simulink model "flightController"  (R2021a)
settings: Solver=ode3  StartTime=0  StopTime=10  FixedStep=Ts  RelTol=1e-3  EnableMultiTasking=on
undefined symbols (not defined in the file): Controller, ControlvsRed, D_ROLL, delays, DiscIntNeverNeededParam, g, I_ROLL, norm_act, Normalization, P_Pitch, P_ROLL, P_Roll, P_Yaw, P_z, PR_Start, save_time, sts_cnames, time_DisYaw, time_stepsX, time_stepsY, time_stepsZ, Ts, Vehicle, x0, x0_f
libraries: deeplib x5
(part 2 of 4)

== system flightController/Flight Controller/Perturbaciones/Perturbaciones en Pitch ==
  Add : Sum  Inputs=++++++++
  Pulse Generator1 : DiscretePulseGenerator  PulseType=Time based  Amplitude=P_Pitch(2)  Period=150  PulseWidth=0.01  PhaseDelay=time_stepsX(2)
  Pulse Generator2 : DiscretePulseGenerator  PulseType=Time based  Amplitude=P_Pitch(1)  Period=150  PulseWidth=0.02  PhaseDelay=time_stepsX(1)
  Pulse Generator3 : DiscretePulseGenerator  PulseType=Time based  Amplitude=P_Pitch(3)  Period=150  PulseWidth=0.01  PhaseDelay=time_stepsX(3)
  Pulse Generator4 : DiscretePulseGenerator  PulseType=Time based  Amplitude=P_Pitch(4)  Period=150  PulseWidth=0.01  PhaseDelay=time_stepsX(4)
  Pulse Generator5 : DiscretePulseGenerator  PulseType=Time based  Amplitude=P_Pitch(5)  Period=1500  PulseWidth=0.001  PhaseDelay=time_stepsX(5)
  Pulse Generator6 : DiscretePulseGenerator  PulseType=Time based  Amplitude=P_Pitch(6)  Period=150  PulseWidth=0.01  PhaseDelay=time_stepsX(6)
  Pulse Generator7 : DiscretePulseGenerator  PulseType=Time based  Amplitude=P_Pitch(7)  Period=1500  PulseWidth=0.001  PhaseDelay=time_stepsX(7)
  Pulse Generator8 : DiscretePulseGenerator  PulseType=Time based  Amplitude=P_Pitch(8)  Period=1500  PulseWidth=0.001  PhaseDelay=time_stepsX(8)
  Out1 : Outport
  wires:
  Pulse Generator2/1 -> Add/1
  Pulse Generator1/1 -> Add/2
  Pulse Generator3/1 -> Add/3
  Pulse Generator4/1 -> Add/4
  Pulse Generator5/1 -> Add/5
  Add/1 -> Out1/1
  Pulse Generator6/1 -> Add/6
  Pulse Generator7/1 -> Add/7
  Pulse Generator8/1 -> Add/8

== system flightController/Flight Controller/Perturbaciones/Perturbaciones en Roll ==
  Add : Sum  Inputs=++++++++
  Add1 : Sum  Commented=on  Inputs=+++++++
  Pulse Generator1 : DiscretePulseGenerator  PulseType=Time based  Amplitude=P_Roll(2)  Period=1500  PulseWidth=0.001  PhaseDelay=time_stepsY(2)
  Pulse Generator10 : DiscretePulseGenerator  Commented=on  PulseType=Time based  Amplitude=P_Roll(3)  Period=1500  PulseWidth=0.001  PhaseDelay=35
  Pulse Generator11 : DiscretePulseGenerator  Commented=on  PulseType=Time based  Amplitude=P_Roll(4)  Period=1500  PulseWidth=0.001  PhaseDelay=50
  Pulse Generator12 : DiscretePulseGenerator  Commented=on  PulseType=Time based  Amplitude=P_Roll(5)  Period=1500  PulseWidth=0.001  PhaseDelay=75
  Pulse Generator13 : DiscretePulseGenerator  Commented=on  PulseType=Time based  Amplitude=P_Roll(6)  Period=1500  PulseWidth=0.001  PhaseDelay=90
  Pulse Generator14 : DiscretePulseGenerator  Commented=on  PulseType=Time based  Amplitude=P_Roll(2)  Period=1500  PulseWidth=0.001  PhaseDelay=90
  Pulse Generator15 : DiscretePulseGenerator  PulseType=Time based  Amplitude=P_Roll(8)  Period=1500  PulseWidth=0.001  PhaseDelay=PR_Start
  Pulse Generator2 : DiscretePulseGenerator  PulseType=Time based  Amplitude=P_Roll(1)  Period=1500  PulseWidth=0.001  PhaseDelay=time_stepsY(1)
  Pulse Generator3 : DiscretePulseGenerator  PulseType=Time based  Amplitude=P_Roll(3)  Period=1500  PulseWidth=0.001  PhaseDelay=time_stepsY(3)
  Pulse Generator4 : DiscretePulseGenerator  PulseType=Time based  Amplitude=P_Roll(4)  Period=1500  PulseWidth=0.001  PhaseDelay=time_stepsY(4)
  Pulse Generator5 : DiscretePulseGenerator  PulseType=Time based  Amplitude=P_Roll(5)  Period=1500  PulseWidth=0.001  PhaseDelay=time_stepsY(5)
  Pulse Generator6 : DiscretePulseGenerator  PulseType=Time based  Amplitude=P_Roll(6)  Period=1500  PulseWidth=0.001  PhaseDelay=time_stepsY(6)
  Pulse Generator7 : DiscretePulseGenerator  PulseType=Time based  Amplitude=P_Roll(7)  Period=1500  PulseWidth=0.001  PhaseDelay=time_stepsY(7)
  Pulse Generator8 : DiscretePulseGenerator  Commented=on  PulseType=Time based  Amplitude=P_Roll(2)  Period=1500  PulseWidth=0.001  PhaseDelay=20
  Pulse Generator9 : DiscretePulseGenerator  Commented=on  PulseType=Time based  Amplitude=P_Roll(1)  Period=1500  PulseWidth=0.001  PhaseDelay=5
  Scope : Scope
  Out1 : Outport
  wires:
  Add/1 -> Out1/1
  Pulse Generator14/1 -> Add1/7
  Pulse Generator12/1 -> Add1/5
  Pulse Generator8/1 -> Add1/2
  Pulse Generator10/1 -> Add1/3
  Pulse Generator13/1 -> Add1/6
  Pulse Generator9/1 -> Add1/1
  Pulse Generator11/1 -> Add1/4
  Pulse Generator2/1 -> Add/2
  Pulse Generator1/1 -> Add/3
  Pulse Generator3/1 -> Add/4
  Pulse Generator4/1 -> Add/5
  Pulse Generator5/1 -> Add/6
  Pulse Generator6/1 -> Add/7
  Pulse Generator7/1 -> Add/8
  Pulse Generator15/1 -> Scope/1, Add/1

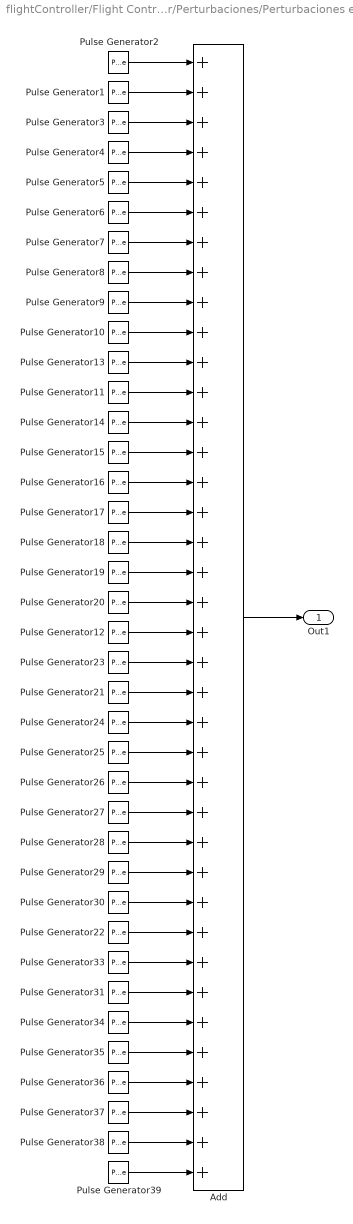
== system flightController/Flight Controller/Perturbaciones/Perturbaciones en Yaw ==
  Add : Sum  Inputs=++++++++++++++++++++++++++++++++++++++
  Pulse Generator1 : DiscretePulseGenerator  PulseType=Time based  Amplitude=P_Yaw(2)  Period=150  PulseWidth=0.01  PhaseDelay=time_DisYaw(2)
  Pulse Generator10 : DiscretePulseGenerator  PulseType=Time based  Amplitude=P_Yaw(10)  Period=1500  PulseWidth=0.001  PhaseDelay=time_DisYaw(10)
  Pulse Generator11 : DiscretePulseGenerator  PulseType=Time based  Amplitude=P_Yaw(12)  Period=150  PulseWidth=0.01  PhaseDelay=time_DisYaw(11)
  Pulse Generator12 : DiscretePulseGenerator  PulseType=Time based  Amplitude=P_Yaw(20)  Period=1500  PulseWidth=0.001  PhaseDelay=time_DisYaw(20)
  Pulse Generator13 : DiscretePulseGenerator  PulseType=Time based  Amplitude=P_Yaw(11)  Period=150  PulseWidth=0.02  PhaseDelay=time_DisYaw(11)
  Pulse Generator14 : DiscretePulseGenerator  PulseType=Time based  Amplitude=P_Yaw(13)  Period=150  PulseWidth=0.01  PhaseDelay=time_DisYaw(13)
  Pulse Generator15 : DiscretePulseGenerator  PulseType=Time based  Amplitude=P_Yaw(14)  Period=150  PulseWidth=0.01  PhaseDelay=time_DisYaw(14)
  Pulse Generator16 : DiscretePulseGenerator  PulseType=Time based  Amplitude=P_Yaw(15)  Period=1500  PulseWidth=0.001  PhaseDelay=time_DisYaw(15)
  Pulse Generator17 : DiscretePulseGenerator  PulseType=Time based  Amplitude=P_Yaw(16)  Period=150  PulseWidth=0.01  PhaseDelay=time_DisYaw(16)
  Pulse Generator18 : DiscretePulseGenerator  PulseType=Time based  Amplitude=P_Yaw(17)  Period=1500  PulseWidth=0.001  PhaseDelay=time_DisYaw(17)
  Pulse Generator19 : DiscretePulseGenerator  PulseType=Time based  Amplitude=P_Yaw(18)  Period=1500  PulseWidth=0.001  PhaseDelay=time_DisYaw(18)
  Pulse Generator2 : DiscretePulseGenerator  PulseType=Time based  Amplitude=P_Yaw(1)  Period=150  PulseWidth=0.02  PhaseDelay=time_DisYaw(1)
  Pulse Generator20 : DiscretePulseGenerator  PulseType=Time based  Amplitude=P_Yaw(19)  Period=1500  PulseWidth=0.001  PhaseDelay=time_DisYaw(19)
  Pulse Generator21 : DiscretePulseGenerator  PulseType=Time based  Amplitude=P_Yaw(22)  Period=150  PulseWidth=0.01  PhaseDelay=time_DisYaw(22)
  Pulse Generator22 : DiscretePulseGenerator  PulseType=Time based  Amplitude=P_Yaw(30)  Period=1500  PulseWidth=0.001  PhaseDelay=time_DisYaw(30)
  Pulse Generator23 : DiscretePulseGenerator  PulseType=Time based  Amplitude=P_Yaw(21)  Period=150  PulseWidth=0.02  PhaseDelay=time_DisYaw(21)
  Pulse Generator24 : DiscretePulseGenerator  PulseType=Time based  Amplitude=P_Yaw(23)  Period=150  PulseWidth=0.01  PhaseDelay=time_DisYaw(22)
  Pulse Generator25 : DiscretePulseGenerator  PulseType=Time based  Amplitude=P_Yaw(24)  Period=150  PulseWidth=0.01  PhaseDelay=time_DisYaw(24)
  Pulse Generator26 : DiscretePulseGenerator  PulseType=Time based  Amplitude=P_Yaw(25)  Period=1500  PulseWidth=0.001  PhaseDelay=time_DisYaw(25)
  Pulse Generator27 : DiscretePulseGenerator  PulseType=Time based  Amplitude=P_Yaw(26)  Period=150  PulseWidth=0.01  PhaseDelay=time_DisYaw(26)
  Pulse Generator28 : DiscretePulseGenerator  PulseType=Time based  Amplitude=P_Yaw(27)  Period=1500  PulseWidth=0.001  PhaseDelay=time_DisYaw(27)
  Pulse Generator29 : DiscretePulseGenerator  PulseType=Time based  Amplitude=P_Yaw(28)  Period=1500  PulseWidth=0.001  PhaseDelay=time_DisYaw(28)
  Pulse Generator3 : DiscretePulseGenerator  PulseType=Time based  Amplitude=P_Yaw(3)  Period=150  PulseWidth=0.01  PhaseDelay=time_DisYaw(3)
  Pulse Generator30 : DiscretePulseGenerator  PulseType=Time based  Amplitude=P_Yaw(29)  Period=1500  PulseWidth=0.001  PhaseDelay=time_DisYaw(29)
  Pulse Generator31 : DiscretePulseGenerator  PulseType=Time based  Amplitude=P_Yaw(32)  Period=150  PulseWidth=0.01  PhaseDelay=time_DisYaw(32)
  Pulse Generator33 : DiscretePulseGenerator  PulseType=Time based  Amplitude=P_Yaw(31)  Period=150  PulseWidth=0.02  PhaseDelay=time_DisYaw(31)
  Pulse Generator34 : DiscretePulseGenerator  PulseType=Time based  Amplitude=P_Yaw(33)  Period=150  PulseWidth=0.01  PhaseDelay=time_DisYaw(33)
  Pulse Generator35 : DiscretePulseGenerator  PulseType=Time based  Amplitude=P_Yaw(34)  Period=150  PulseWidth=0.01  PhaseDelay=time_DisYaw(34)
  Pulse Generator36 : DiscretePulseGenerator  PulseType=Time based  Amplitude=P_Yaw(35)  Period=1500  PulseWidth=0.001  PhaseDelay=time_DisYaw(35)
  Pulse Generator37 : DiscretePulseGenerator  PulseType=Time based  Amplitude=P_Yaw(36)  Period=150  PulseWidth=0.01  PhaseDelay=time_DisYaw(36)
  Pulse Generator38 : DiscretePulseGenerator  PulseType=Time based  Amplitude=P_Yaw(37)  Period=1500  PulseWidth=0.001  PhaseDelay=time_DisYaw(37)
  Pulse Generator39 : DiscretePulseGenerator  PulseType=Time based  Amplitude=P_Yaw(38)  Period=1500  PulseWidth=0.001  PhaseDelay=time_DisYaw(38)
  Pulse Generator4 : DiscretePulseGenerator  PulseType=Time based  Amplitude=P_Yaw(4)  Period=150  PulseWidth=0.01  PhaseDelay=time_DisYaw(4)
  Pulse Generator5 : DiscretePulseGenerator  PulseType=Time based  Amplitude=P_Yaw(5)  Period=1500  PulseWidth=0.001  PhaseDelay=time_DisYaw(5)
  Pulse Generator6 : DiscretePulseGenerator  PulseType=Time based  Amplitude=P_Yaw(6)  Period=150  PulseWidth=0.01  PhaseDelay=time_DisYaw(6)
  Pulse Generator7 : DiscretePulseGenerator  PulseType=Time based  Amplitude=P_Yaw(7)  Period=1500  PulseWidth=0.001  PhaseDelay=time_DisYaw(7)
  Pulse Generator8 : DiscretePulseGenerator  PulseType=Time based  Amplitude=P_Yaw(8)  Period=1500  PulseWidth=0.001  PhaseDelay=time_DisYaw(8)
  Pulse Generator9 : DiscretePulseGenerator  PulseType=Time based  Amplitude=P_Yaw(9)  Period=1500  PulseWidth=0.001  PhaseDelay=time_DisYaw(9)
  Out1 : Outport
  wires:
  Pulse Generator8/1 -> Add/8
  Pulse Generator7/1 -> Add/7
  Pulse Generator6/1 -> Add/6
  Add/1 -> Out1/1
  Pulse Generator5/1 -> Add/5
  Pulse Generator4/1 -> Add/4
  Pulse Generator3/1 -> Add/3
  Pulse Generator1/1 -> Add/2
  Pulse Generator2/1 -> Add/1
  Pulse Generator9/1 -> Add/9
  Pulse Generator10/1 -> Add/10
  Pulse Generator12/1 -> Add/20
  Pulse Generator13/1 -> Add/11
  Pulse Generator16/1 -> Add/15
  Pulse Generator11/1 -> Add/12
  Pulse Generator20/1 -> Add/19
  Pulse Generator19/1 -> Add/18
  Pulse Generator18/1 -> Add/17
  Pulse Generator15/1 -> Add/14
  Pulse Generator14/1 -> Add/13
  Pulse Generator17/1 -> Add/16
  Pulse Generator22/1 -> Add/30
  Pulse Generator23/1 -> Add/21
  Pulse Generator26/1 -> Add/25
  Pulse Generator21/1 -> Add/22
  Pulse Generator30/1 -> Add/29
  Pulse Generator29/1 -> Add/28
  Pulse Generator28/1 -> Add/27
  Pulse Generator25/1 -> Add/24
  Pulse Generator24/1 -> Add/23
  Pulse Generator27/1 -> Add/26
  Pulse Generator33/1 -> Add/31
  Pulse Generator36/1 -> Add/35
  Pulse Generator31/1 -> Add/32
  Pulse Generator39/1 -> Add/38
  Pulse Generator38/1 -> Add/37
  Pulse Generator35/1 -> Add/34
  Pulse Generator34/1 -> Add/33
  Pulse Generator37/1 -> Add/36

== system flightController/Flight Controller/Perturbaciones/Perturbaciones en Z ==
  Add : Sum  Inputs=++++++++++++++++++++
  Pulse Generator1 : DiscretePulseGenerator  PulseType=Time based  Amplitude=P_z(2)  Period=150  PulseWidth=0.5  PhaseDelay=time_stepsZ(2)
  Pulse Generator10 : DiscretePulseGenerator  PulseType=Time based  Amplitude=P_z(10)  Period=150  PulseWidth=0.5  PhaseDelay=time_stepsZ(10)
  Pulse Generator11 : DiscretePulseGenerator  PulseType=Time based  Amplitude=P_z(11)  Period=150  PulseWidth=0.5  PhaseDelay=time_stepsZ(11)
  Pulse Generator12 : DiscretePulseGenerator  PulseType=Time based  Amplitude=P_z(12)  Period=150  PulseWidth=0.5  PhaseDelay=time_stepsZ(12)
  Pulse Generator13 : DiscretePulseGenerator  PulseType=Time based  Amplitude=P_z(13)  Period=150  PulseWidth=0.5  PhaseDelay=time_stepsZ(13)
  Pulse Generator14 : DiscretePulseGenerator  PulseType=Time based  Amplitude=P_z(14)  Period=150  PulseWidth=0.5  PhaseDelay=time_stepsZ(14)
  Pulse Generator15 : DiscretePulseGenerator  PulseType=Time based  Amplitude=P_z(15)  Period=150  PulseWidth=0.5  PhaseDelay=time_stepsZ(15)
  Pulse Generator16 : DiscretePulseGenerator  PulseType=Time based  Amplitude=P_z(16)  Period=150  PulseWidth=0.2  PhaseDelay=time_stepsZ(16)
  Pulse Generator17 : DiscretePulseGenerator  PulseType=Time based  Amplitude=P_z(17)  Period=150  PulseWidth=0.3  PhaseDelay=time_stepsZ(17)
  Pulse Generator18 : DiscretePulseGenerator  PulseType=Time based  Amplitude=P_z(18)  Period=150  PulseWidth=0.1  PhaseDelay=time_stepsZ(18)
  Pulse Generator19 : DiscretePulseGenerator  PulseType=Time based  Amplitude=P_z(19)  Period=150  PulseWidth=0.5  PhaseDelay=time_stepsZ(19)
  Pulse Generator2 : DiscretePulseGenerator  PulseType=Time based  Amplitude=P_z(1)  Period=150  PulseWidth=0.5  PhaseDelay=time_stepsZ(1)
  Pulse Generator20 : DiscretePulseGenerator  PulseType=Time based  Amplitude=P_z(20)  Period=150  PulseWidth=0.01  PhaseDelay=time_stepsZ(20)
  Pulse Generator3 : DiscretePulseGenerator  PulseType=Time based  Amplitude=P_z(3)  Period=150  PulseWidth=0.5  PhaseDelay=time_stepsZ(3)
  Pulse Generator4 : DiscretePulseGenerator  PulseType=Time based  Amplitude=P_z(4)  Period=150  PulseWidth=0.5  PhaseDelay=time_stepsZ(4)
  Pulse Generator5 : DiscretePulseGenerator  PulseType=Time based  Amplitude=P_z(5)  Period=150  PulseWidth=0.5  PhaseDelay=time_stepsZ(5)
  Pulse Generator6 : DiscretePulseGenerator  PulseType=Time based  Amplitude=P_z(6)  Period=150  PulseWidth=0.5  PhaseDelay=time_stepsZ(6)
  Pulse Generator7 : DiscretePulseGenerator  PulseType=Time based  Amplitude=P_z(7)  Period=150  PulseWidth=0.5  PhaseDelay=time_stepsZ(7)
  Pulse Generator8 : DiscretePulseGenerator  PulseType=Time based  Amplitude=P_z(8)  Period=150  PulseWidth=0.5  PhaseDelay=time_stepsZ(8)
  Pulse Generator9 : DiscretePulseGenerator  PulseType=Time based  Amplitude=P_z(9)  Period=150  PulseWidth=0.5  PhaseDelay=time_stepsZ(9)
  Out1 : Outport
  wires:
  Pulse Generator2/1 -> Add/1
  Pulse Generator1/1 -> Add/2
  Pulse Generator3/1 -> Add/3
  Pulse Generator4/1 -> Add/4
  Pulse Generator5/1 -> Add/5
  Add/1 -> Out1/1
  Pulse Generator6/1 -> Add/6
  Pulse Generator7/1 -> Add/7
  Pulse Generator8/1 -> Add/8
  Pulse Generator9/1 -> Add/9
  Pulse Generator10/1 -> Add/10
  Pulse Generator11/1 -> Add/11
  Pulse Generator12/1 -> Add/12
  Pulse Generator13/1 -> Add/13
  Pulse Generator14/1 -> Add/14
  Pulse Generator15/1 -> Add/15
  Pulse Generator16/1 -> Add/16
  Pulse Generator17/1 -> Add/17
  Pulse Generator18/1 -> Add/18
  Pulse Generator19/1 -> Add/19
  Pulse Generator20/1 -> Add/20

== system flightController/Variant Subsystem/ANN/Subsystem ==
  Referencia : Inport
  Pos_estim : Inport  Port=2
  Sensores : Inport  Port=3  OutDataTypeStr=Bus: sensordata_t
  Math Function : Math  Commented=on  Operator=transpose  SaturateOnIntegerOverflow=on
  Mux : Mux  Inputs=5
  Subsystem : Subsystem
  Subsystem10 : Subsystem  Commented=on
  Subsystem11 : Subsystem  Commented=on
  Subsystem12 : Subsystem  Commented=on
  Subsystem13 : Subsystem
  Subsystem3 : Subsystem
  Norm_States : Outport
  wires:
  Mux/1 -> Norm_States/1
  Pos_estim/1 -> Subsystem13/1(In1)
  Subsystem13/1(Pos_Norm) -> Mux/1
  Referencia/1 -> Subsystem3/1(In1)
  Subsystem3/1(Z_r) -> Mux/2
  Subsystem3/2(Dz_r) -> Mux/3
  Sensores/1 -> Subsystem/1(In1)
  Subsystem13/2(Acceleracion Pos) -> Mux/5
  Subsystem/1(Ac_Dz) -> Mux/4

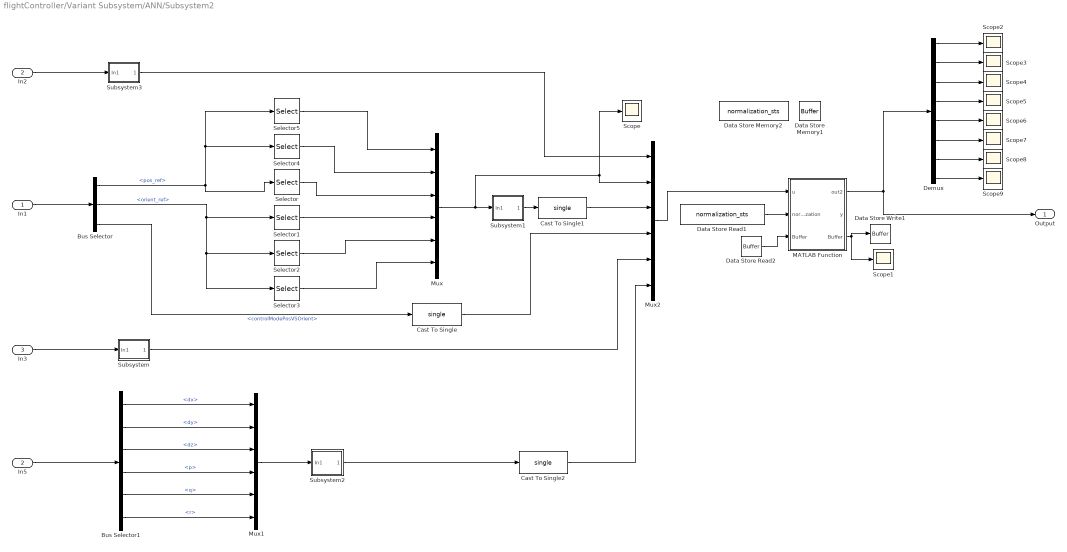
== system flightController/Variant Subsystem/ANN/Subsystem2 ==
  In1 : Inport
  In2 : Inport  Port=2
  In3 : Inport  Port=3
  Bus Selector : BusSelector  OutputSignals=pos_ref,orient_ref,controlModePosVSOrient
  Bus Selector1 : BusSelector  OutputSignals=dx,dy,dz,p,q,r
  Cast To Single : DataTypeConversion  OutDataTypeStr=single
  Cast To Single1 : DataTypeConversion  OutDataTypeStr=single
  Cast To Single2 : DataTypeConversion  OutDataTypeStr=single
  Data Store Memory1 : DataStoreMemory  DataStoreName=Buffer  ReadBeforeWriteMsg=warning  WriteAfterWriteMsg=warning  WriteAfterReadMsg=warning  InitialValue=repmat(x0,1,delays+1)  ShowAdditionalParam=off
  Data Store Memory2 : DataStoreMemory  DataStoreName=normalization_sts  ReadBeforeWriteMsg=warning  WriteAfterWriteMsg=warning  WriteAfterReadMsg=warning  InitialValue=normalization_sts  ShowAdditionalParam=off
  Data Store Read1 : DataStoreRead  DataStoreName=normalization_sts  IndexOptions=Index vector (dialog)  Indices=1  OutputSizes=1
  Data Store Read2 : DataStoreRead  DataStoreName=Buffer  IndexOptions=Index vector (dialog)  Indices=1  OutputSizes=1
  Data Store Write1 : DataStoreWrite  DataStoreName=Buffer  IndexOptions=Index vector (dialog)  Indices=1  OutputSizes=1
  Demux : Demux  Outputs=8
  In5 : InportShadow  Port=2
  MATLAB Function : MATLAB Function  TreatAsAtomicUnit=on
  Mux : Mux  Inputs=6
  Mux1 : Mux  Inputs=6
  Mux2 : Mux  Inputs=6
      settings: DisplayOption=signals
  Scope{,1..9} (10 alike) : Scope
  Selector : Selector  InputPortWidth=3  IndexOptions=Index vector (dialog)  Indices=[3]  OutputSizes=1
  Selector1 : Selector  InputPortWidth=3  IndexOptions=Index vector (dialog)  Indices=[1]  OutputSizes=1
  Selector2 : Selector  InputPortWidth=3  IndexOptions=Index vector (dialog)  Indices=[3]  OutputSizes=1
  Selector3 : Selector  InputPortWidth=3  IndexOptions=Index vector (dialog)  Indices=[2]  OutputSizes=1
  Selector4 : Selector  InputPortWidth=3  IndexOptions=Index vector (dialog)  Indices=[2]  OutputSizes=1
  Selector5 : Selector  InputPortWidth=3  IndexOptions=Index vector (dialog)  Indices=[1]  OutputSizes=1
  Subsystem : Subsystem
  Subsystem1 : Subsystem
  Subsystem2 : Subsystem
  Subsystem3 : Subsystem
  Output : Outport
  wires:
  In1/1 -> Bus Selector/1
  Bus Selector/2 -> Selector3/1, Selector2/1, Selector1/1  "<orient_ref>"
  Bus Selector/1 -> Selector/1, Selector5/1, Selector4/1  "<pos_ref>"
  Selector5/1 -> Mux/1
  Selector4/1 -> Mux/2
  Selector/1 -> Mux/3
  Selector1/1 -> Mux/4
  Selector2/1 -> Mux/5
  Selector3/1 -> Mux/6
  Mux/1 -> Mux2/2, Scope/1, Subsystem1/1(In1)
  In5/1 -> Bus Selector1/1
  Bus Selector1/1 -> Mux1/1  "<dx>"
  Bus Selector1/2 -> Mux1/2  "<dy>"
  Bus Selector1/3 -> Mux1/3  "<dz>"
  Bus Selector1/4 -> Mux1/4  "<p>"
  Bus Selector1/5 -> Mux1/5  "<q>"
  Bus Selector1/6 -> Mux1/6  "<r>"
  Mux1/1 -> Subsystem2/1(In1)
  Mux2/1 -> MATLAB Function/1(u)
  In3/1 -> Subsystem/1(In1)
  In2/1 -> Subsystem3/1(In1)
  Bus Selector/3 -> Cast To Single/1  "<controlModePosVSOrient>"
  Cast To Single1/1 -> Mux2/3
  Subsystem1/1(Out1) -> Cast To Single1/1
  Subsystem2/1(Out1) -> Cast To Single2/1
  Data Store Read1/1 -> MATLAB Function/2(normalization)
  Data Store Read2/1 -> MATLAB Function/3("Buffer ")
  MATLAB Function/3(Buffer) -> Data Store Write1/1, Scope1/1
  Subsystem3/1(Out5) -> Mux2/1
  Cast To Single2/1 -> Mux2/6
  Subsystem/1(Out5) -> Mux2/5
  Cast To Single/1 -> Mux2/4
  MATLAB Function/1(out2) -> Output/1, Demux/1
  Demux/1 -> Scope2/1
  Demux/2 -> Scope3/1
  Demux/3 -> Scope4/1
  Demux/4 -> Scope5/1
  Demux/5 -> Scope6/1
  Demux/6 -> Scope7/1
  Demux/7 -> Scope8/1
  Demux/8 -> Scope9/1

== system flightController/Variant Subsystem/ANN/Subsystem3 ==
  In1 : Inport
  Constant : Constant  Value=norm_act(1)
  Constant1 : Constant  Value=norm_act(3)
  Constant2 : Constant  Value=norm_act(5)
  Constant3 : Constant  Value=norm_act(7)
  Data Type Conversion : DataTypeConversion  OutDataTypeStr=single
  Demux : Demux
  Gain : Gain  Gain=(norm_act(2)-norm_act(1))  ParamDataTypeStr=single  OutDataTypeStr=single
  Gain1 : Gain  Gain=(norm_act(4)-norm_act(3))  OutDataTypeStr=single
  Gain2 : Gain  Gain=(norm_act(6)-norm_act(5))  OutDataTypeStr=single
  Gain3 : Gain  Gain=(norm_act(8)-norm_act(7))  OutDataTypeStr=single
  Mux : Mux
  Scope{,1..7} (8 alike) : Scope
  Sum{,1..3} (4 alike) : Sum  Inputs=|++
  motors_refout : Outport
  wires:
  In1/1 -> Demux/1
  Demux/4 -> Scope5/1, Gain3/1
  Constant/1 -> Sum/2
  Gain/1 -> Sum/1
  Demux/1 -> Scope4/1, Gain/1
  Gain1/1 -> Sum1/1
  Constant1/1 -> Sum1/2
  Demux/2 -> Gain1/1, Scope6/1
  Gain2/1 -> Sum2/1
  Constant2/1 -> Sum2/2
  Demux/3 -> Scope7/1, Gain2/1
  Gain3/1 -> Sum3/1
  Constant3/1 -> Sum3/2
  Mux/1 -> Data Type Conversion/1
  Data Type Conversion/1 -> motors_refout/1
  Sum3/1 -> Mux/4, Scope3/1
  Sum1/1 -> Mux/2, Scope1/1
  Sum/1 -> Mux/1, Scope/1
  Sum2/1 -> Mux/3, Scope2/1

== system flightController/Variant Subsystem/ANN/Subsystem4 ==
  In1 : Inport
  Constant : Constant  Value=norm_act(1)
  Constant1 : Constant  Value=norm_act(3)
  Constant2 : Constant  Value=norm_act(5)
  Constant3 : Constant  Value=norm_act(7)
  Data Type Conversion : DataTypeConversion  OutDataTypeStr=single
  Demux : Demux
  Gain : Gain  Gain=(norm_act(2)-norm_act(1))
  Gain1 : Gain  Gain=(norm_act(4)-norm_act(3))
  Gain2 : Gain  Gain=(norm_act(6)-norm_act(5))
  Gain3 : Gain  Gain=(norm_act(8)-norm_act(7))
  Mux : Mux
  Scope{,1..7} (8 alike) : Scope
  Sum{,1..3} (4 alike) : Sum  Inputs=|++
  motors_refout : Outport
  wires:
  In1/1 -> Demux/1
  Demux/4 -> Scope5/1, Gain3/1
  Constant/1 -> Sum/2
  Gain/1 -> Sum/1
  Demux/1 -> Scope4/1, Gain/1
  Gain1/1 -> Sum1/1
  Constant1/1 -> Sum1/2
  Demux/2 -> Gain1/1, Scope6/1
  Gain2/1 -> Sum2/1
  Constant2/1 -> Sum2/2
  Demux/3 -> Scope7/1, Gain2/1
  Gain3/1 -> Sum3/1
  Constant3/1 -> Sum3/2
  Mux/1 -> Data Type Conversion/1
  Data Type Conversion/1 -> motors_refout/1
  Sum3/1 -> Mux/4, Scope3/1
  Sum1/1 -> Mux/2, Scope1/1
  Sum/1 -> Mux/1, Scope/1
  Sum2/1 -> Mux/3, Scope2/1

== system flightController/Variant Subsystem/ANN_Feedback/Subsystem ==
  In1 : Inport
  Constant : Constant  Value=norm_act(1)
  Constant1 : Constant  Value=norm_act(3)
  Constant2 : Constant  Value=norm_act(5)
  Constant3 : Constant  Value=norm_act(7)
  Demux : Demux
  Gain1 : Gain  Gain=1/(norm_act(2)-norm_act(1))
  Gain2 : Gain  Gain=1/(norm_act(4)-norm_act(3))
  Gain3 : Gain  Gain=1/(norm_act(6)-norm_act(5))
  Gain4 : Gain  Gain=1/(norm_act(8)-norm_act(7))
  Mux : Mux
  Sum{,1..3} (4 alike) : Sum  Inputs=|+-
  Out1 : Outport
  wires:
  Sum/1 -> Gain1/1
  Demux/1 -> Sum/1
  Constant/1 -> Sum/2
  In1/1 -> Demux/1
  Sum1/1 -> Gain2/1
  Constant1/1 -> Sum1/2
  Demux/2 -> Sum1/1
  Demux/3 -> Sum2/1
  Constant2/1 -> Sum2/2
  Sum2/1 -> Gain3/1
  Sum3/1 -> Gain4/1
  Constant3/1 -> Sum3/2
  Demux/4 -> Sum3/1
  Mux/1 -> Out1/1
  Gain1/1 -> Mux/1
  Gain2/1 -> Mux/2
  Gain3/1 -> Mux/3
  Gain4/1 -> Mux/4

== system flightController/Variant Subsystem/ANN_Feedback/Subsystem1 ==
  Referencia : Inport
  Pos_estim : Inport  Port=2
  Sensores : Inport  Port=3  OutDataTypeStr=Bus: sensordata_t
  Math Function : Math  Commented=on  Operator=transpose  SaturateOnIntegerOverflow=on
  Mux : Mux
  Subsystem : Subsystem  Commented=on
  Subsystem10 : Subsystem  Commented=on
  Subsystem11 : Subsystem  Commented=on
  Subsystem12 : Subsystem  Commented=on
  Subsystem13 : Subsystem
  Subsystem3 : Subsystem
  Norm_States : Outport
  wires:
  Mux/1 -> Norm_States/1
  Pos_estim/1 -> Subsystem13/1(In1)
  Subsystem13/1(Pos_Norm) -> Mux/1
  Referencia/1 -> Subsystem3/1(In1)
  Subsystem3/1(Z_r) -> Mux/2
  Subsystem3/2(Dz_r) -> Mux/3
  Sensores/1 -> Subsystem/1(In1)
  Subsystem13/2(Acceleracion Pos) -> Mux/4

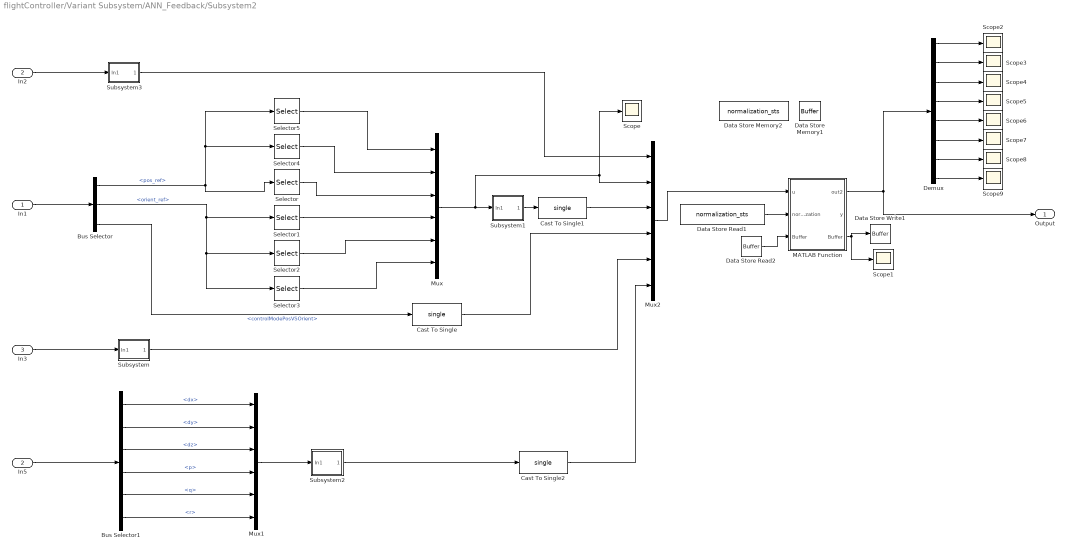
== system flightController/Variant Subsystem/ANN_Feedback/Subsystem2 ==
  In1 : Inport
  In2 : Inport  Port=2
  In3 : Inport  Port=3
  Bus Selector : BusSelector  OutputSignals=pos_ref,orient_ref,controlModePosVSOrient
  Bus Selector1 : BusSelector  OutputSignals=dx,dy,dz,p,q,r
  Cast To Single : DataTypeConversion  OutDataTypeStr=single
  Cast To Single1 : DataTypeConversion  OutDataTypeStr=single
  Cast To Single2 : DataTypeConversion  OutDataTypeStr=single
  Data Store Memory1 : DataStoreMemory  DataStoreName=Buffer  ReadBeforeWriteMsg=warning  WriteAfterWriteMsg=warning  WriteAfterReadMsg=warning  InitialValue=repmat(x0,1,delays+1)  ShowAdditionalParam=off
  Data Store Memory2 : DataStoreMemory  DataStoreName=normalization_sts  ReadBeforeWriteMsg=warning  WriteAfterWriteMsg=warning  WriteAfterReadMsg=warning  InitialValue=normalization_sts  ShowAdditionalParam=off
  Data Store Read1 : DataStoreRead  DataStoreName=normalization_sts  IndexOptions=Index vector (dialog)  Indices=1  OutputSizes=1
  Data Store Read2 : DataStoreRead  DataStoreName=Buffer  IndexOptions=Index vector (dialog)  Indices=1  OutputSizes=1
  Data Store Write1 : DataStoreWrite  DataStoreName=Buffer  IndexOptions=Index vector (dialog)  Indices=1  OutputSizes=1
  Demux : Demux  Outputs=8
  In5 : InportShadow  Port=2
  MATLAB Function : MATLAB Function  TreatAsAtomicUnit=on
  Mux : Mux  Inputs=6
  Mux1 : Mux  Inputs=6
  Mux2 : Mux  Inputs=6
      settings: DisplayOption=signals
  Scope{,1..9} (10 alike) : Scope
  Selector : Selector  InputPortWidth=3  IndexOptions=Index vector (dialog)  Indices=[3]  OutputSizes=1
  Selector1 : Selector  InputPortWidth=3  IndexOptions=Index vector (dialog)  Indices=[1]  OutputSizes=1
  Selector2 : Selector  InputPortWidth=3  IndexOptions=Index vector (dialog)  Indices=[3]  OutputSizes=1
  Selector3 : Selector  InputPortWidth=3  IndexOptions=Index vector (dialog)  Indices=[2]  OutputSizes=1
  Selector4 : Selector  InputPortWidth=3  IndexOptions=Index vector (dialog)  Indices=[2]  OutputSizes=1
  Selector5 : Selector  InputPortWidth=3  IndexOptions=Index vector (dialog)  Indices=[1]  OutputSizes=1
  Subsystem : Subsystem
  Subsystem1 : Subsystem
  Subsystem2 : Subsystem
  Subsystem3 : Subsystem
  Output : Outport
  wires:
  In1/1 -> Bus Selector/1
  Bus Selector/2 -> Selector3/1, Selector2/1, Selector1/1  "<orient_ref>"
  Bus Selector/1 -> Selector/1, Selector5/1, Selector4/1  "<pos_ref>"
  Selector5/1 -> Mux/1
  Selector4/1 -> Mux/2
  Selector/1 -> Mux/3
  Selector1/1 -> Mux/4
  Selector2/1 -> Mux/5
  Selector3/1 -> Mux/6
  Mux/1 -> Mux2/2, Scope/1, Subsystem1/1(In1)
  In5/1 -> Bus Selector1/1
  Bus Selector1/1 -> Mux1/1  "<dx>"
  Bus Selector1/2 -> Mux1/2  "<dy>"
  Bus Selector1/3 -> Mux1/3  "<dz>"
  Bus Selector1/4 -> Mux1/4  "<p>"
  Bus Selector1/5 -> Mux1/5  "<q>"
  Bus Selector1/6 -> Mux1/6  "<r>"
  Mux1/1 -> Subsystem2/1(In1)
  Mux2/1 -> MATLAB Function/1(u)
  In3/1 -> Subsystem/1(In1)
  In2/1 -> Subsystem3/1(In1)
  Bus Selector/3 -> Cast To Single/1  "<controlModePosVSOrient>"
  Cast To Single1/1 -> Mux2/3
  Subsystem1/1(Out1) -> Cast To Single1/1
  Subsystem2/1(Out1) -> Cast To Single2/1
  Data Store Read1/1 -> MATLAB Function/2(normalization)
  Data Store Read2/1 -> MATLAB Function/3("Buffer ")
  MATLAB Function/3(Buffer) -> Data Store Write1/1, Scope1/1
  Subsystem3/1(Out5) -> Mux2/1
  Cast To Single2/1 -> Mux2/6
  Subsystem/1(Out5) -> Mux2/5
  Cast To Single/1 -> Mux2/4
  Demux/1 -> Scope2/1
  Demux/2 -> Scope3/1
  Demux/3 -> Scope4/1
  Demux/4 -> Scope5/1
  Demux/5 -> Scope6/1
  Demux/6 -> Scope7/1
  Demux/7 -> Scope8/1
  Demux/8 -> Scope9/1
  MATLAB Function/1(out2) -> Output/1, Demux/1

== system flightController/Variant Subsystem/ANN_Feedback/Subsystem4 ==
  In1 : Inport
  Constant : Constant  Value=norm_act(1)
  Constant1 : Constant  Value=norm_act(3)
  Constant2 : Constant  Value=norm_act(5)
  Constant3 : Constant  Value=norm_act(7)
  Data Type Conversion : DataTypeConversion  OutDataTypeStr=single
  Demux : Demux
  Gain : Gain  Gain=(norm_act(2)-norm_act(1))
  Gain1 : Gain  Gain=(norm_act(4)-norm_act(3))
  Gain2 : Gain  Gain=(norm_act(6)-norm_act(5))
  Gain3 : Gain  Gain=(norm_act(8)-norm_act(7))
  Mux : Mux
  Scope{,1..7} (8 alike) : Scope
  Sum{,1..3} (4 alike) : Sum  Inputs=|++
  motors_refout : Outport
  wires:
  Sum2/1 -> Scope2/1, Mux/3
  Sum/1 -> Scope/1, Mux/1
  Sum1/1 -> Scope1/1, Mux/2
  Sum3/1 -> Scope3/1, Mux/4
  Data Type Conversion/1 -> motors_refout/1
  Mux/1 -> Data Type Conversion/1
  Constant3/1 -> Sum3/2
  Gain3/1 -> Sum3/1
  Demux/3 -> Gain2/1, Scope7/1
  Constant2/1 -> Sum2/2
  Gain2/1 -> Sum2/1
  Demux/2 -> Scope6/1, Gain1/1
  Constant1/1 -> Sum1/2
  Gain1/1 -> Sum1/1
  Demux/1 -> Gain/1, Scope4/1
  Gain/1 -> Sum/1
  Constant/1 -> Sum/2
  Demux/4 -> Gain3/1, Scope5/1
  In1/1 -> Demux/1

== system flightController/Variant Subsystem/ANN_Feedback/Subsystem5 ==
  In1 : Inport
  Constant : Constant  Value=norm_act(1)
  Constant1 : Constant  Value=norm_act(3)
  Constant2 : Constant  Value=norm_act(5)
  Constant3 : Constant  Value=norm_act(7)
  Data Type Conversion : DataTypeConversion  OutDataTypeStr=single
  Demux : Demux
  Gain : Gain  Gain=(norm_act(2)-norm_act(1))
  Gain1 : Gain  Gain=(norm_act(4)-norm_act(3))
  Gain2 : Gain  Gain=(norm_act(6)-norm_act(5))
  Gain3 : Gain  Gain=(norm_act(8)-norm_act(7))
  Mux : Mux
  Scope{,1..7} (8 alike) : Scope
  Sum{,1..3} (4 alike) : Sum  Inputs=|++
  motors_refout : Outport
  wires:
  In1/1 -> Demux/1
  Demux/4 -> Scope5/1, Gain3/1
  Constant/1 -> Sum/2
  Gain/1 -> Sum/1
  Demux/1 -> Scope4/1, Gain/1
  Gain1/1 -> Sum1/1
  Constant1/1 -> Sum1/2
  Demux/2 -> Gain1/1, Scope6/1
  Gain2/1 -> Sum2/1
  Constant2/1 -> Sum2/2
  Demux/3 -> Scope7/1, Gain2/1
  Gain3/1 -> Sum3/1
  Constant3/1 -> Sum3/2
  Mux/1 -> Data Type Conversion/1
  Data Type Conversion/1 -> motors_refout/1
  Sum3/1 -> Mux/4, Scope3/1
  Sum1/1 -> Mux/2, Scope1/1
  Sum/1 -> Mux/1, Scope/1
  Sum2/1 -> Mux/3, Scope2/1

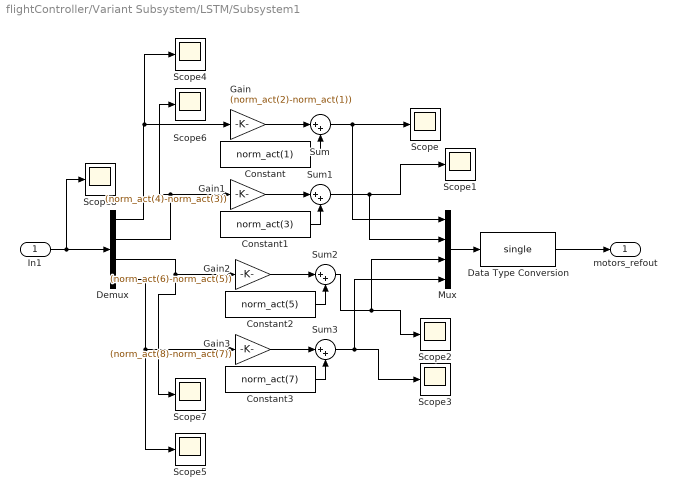
== system flightController/Variant Subsystem/LSTM/Subsystem1 ==
  In1 : Inport
  Constant : Constant  Value=norm_act(1)
  Constant1 : Constant  Value=norm_act(3)
  Constant2 : Constant  Value=norm_act(5)
  Constant3 : Constant  Value=norm_act(7)
  Data Type Conversion : DataTypeConversion  OutDataTypeStr=single
  Demux : Demux
  Gain : Gain  Gain=(norm_act(2)-norm_act(1))
  Gain1 : Gain  Gain=(norm_act(4)-norm_act(3))
  Gain2 : Gain  Gain=(norm_act(6)-norm_act(5))
  Gain3 : Gain  Gain=(norm_act(8)-norm_act(7))
  Mux : Mux
  Scope{,1..8} (9 alike) : Scope
  Sum{,1..3} (4 alike) : Sum  Inputs=|++
  motors_refout : Outport
  wires:
  In1/1 -> Scope8/1, Demux/1
  Demux/4 -> Scope5/1, Gain3/1
  Constant/1 -> Sum/2
  Gain/1 -> Sum/1
  Demux/1 -> Scope4/1, Gain/1
  Gain1/1 -> Sum1/1
  Constant1/1 -> Sum1/2
  Demux/2 -> Gain1/1, Scope6/1
  Gain2/1 -> Sum2/1
  Constant2/1 -> Sum2/2
  Demux/3 -> Scope7/1, Gain2/1
  Gain3/1 -> Sum3/1
  Constant3/1 -> Sum3/2
  Mux/1 -> Data Type Conversion/1
  Data Type Conversion/1 -> motors_refout/1
  Sum3/1 -> Mux/4, Scope3/1
  Sum1/1 -> Mux/2, Scope1/1
  Sum2/1 -> Mux/3, Scope2/1
  Sum/1 -> Mux/1, Scope/1

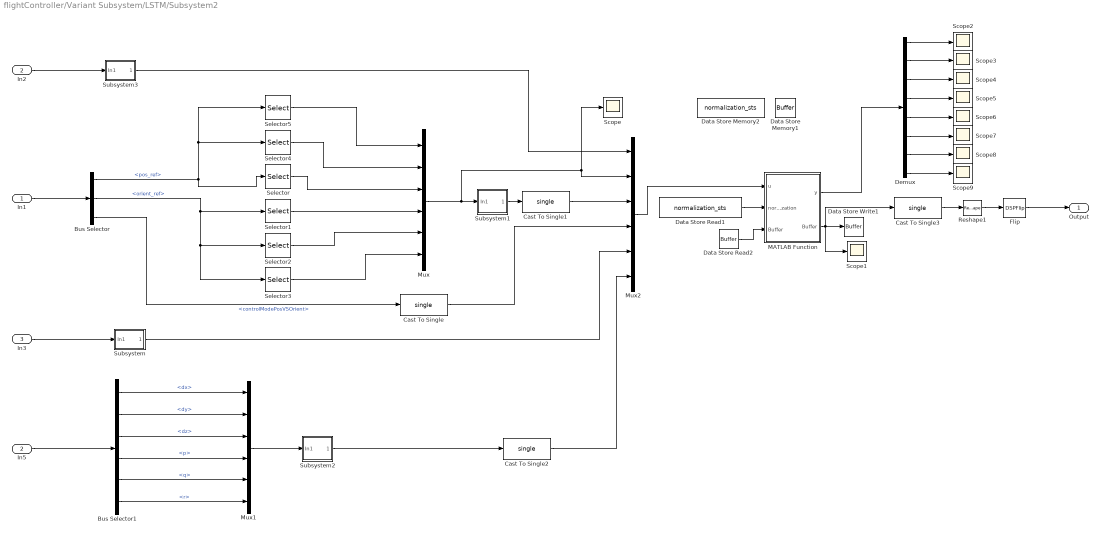
== system flightController/Variant Subsystem/LSTM/Subsystem2 ==
  In1 : Inport
  In2 : Inport  Port=2
  In3 : Inport  Port=3
  Bus Selector : BusSelector  OutputSignals=pos_ref,orient_ref,controlModePosVSOrient
  Bus Selector1 : BusSelector  OutputSignals=dx,dy,dz,p,q,r
  Cast To Single{,1..3} (4 alike) : DataTypeConversion  OutDataTypeStr=single
  Data Store Memory1 : DataStoreMemory  DataStoreName=Buffer  ReadBeforeWriteMsg=warning  WriteAfterWriteMsg=warning  WriteAfterReadMsg=warning  InitialValue=repmat(x0,1,delays+1)  ShowAdditionalParam=off
  Data Store Memory2 : DataStoreMemory  DataStoreName=normalization_sts  ReadBeforeWriteMsg=warning  WriteAfterWriteMsg=warning  WriteAfterReadMsg=warning  InitialValue=normalization_sts  ShowAdditionalParam=off
  Data Store Read1 : DataStoreRead  DataStoreName=normalization_sts  IndexOptions=Index vector (dialog)  Indices=1  OutputSizes=1
  Data Store Read2 : DataStoreRead  DataStoreName=Buffer  IndexOptions=Index vector (dialog)  Indices=1  OutputSizes=1
  Data Store Write1 : DataStoreWrite  DataStoreName=Buffer  IndexOptions=Index vector (dialog)  Indices=1  OutputSizes=1
  Demux : Demux  Outputs=8
  Flip : DSPFlip  dim=Rows
  In5 : InportShadow  Port=2
  MATLAB Function : MATLAB Function  TreatAsAtomicUnit=on
  Mux : Mux  Inputs=6
  Mux1 : Mux  Inputs=6
  Mux2 : Mux  Inputs=6
      settings: DisplayOption=signals
  Reshape1 : Reshape  OutputDimensionality=Customize  OutputDimensions=[length(x0),delays+1]
  Scope{,1..9} (10 alike) : Scope
  Selector : Selector  InputPortWidth=3  IndexOptions=Index vector (dialog)  Indices=[3]  OutputSizes=1
  Selector1 : Selector  InputPortWidth=3  IndexOptions=Index vector (dialog)  Indices=[1]  OutputSizes=1
  Selector2 : Selector  InputPortWidth=3  IndexOptions=Index vector (dialog)  Indices=[3]  OutputSizes=1
  Selector3 : Selector  InputPortWidth=3  IndexOptions=Index vector (dialog)  Indices=[2]  OutputSizes=1
  Selector4 : Selector  InputPortWidth=3  IndexOptions=Index vector (dialog)  Indices=[2]  OutputSizes=1
  Selector5 : Selector  InputPortWidth=3  IndexOptions=Index vector (dialog)  Indices=[1]  OutputSizes=1
  Subsystem : Subsystem
  Subsystem1 : Subsystem
  Subsystem2 : Subsystem
  Subsystem3 : Subsystem
  Output : Outport
  wires:
  In1/1 -> Bus Selector/1
  Bus Selector/2 -> Selector3/1, Selector2/1, Selector1/1  "<orient_ref>"
  Bus Selector/1 -> Selector/1, Selector5/1, Selector4/1  "<pos_ref>"
  Selector5/1 -> Mux/1
  Selector4/1 -> Mux/2
  Selector/1 -> Mux/3
  Selector1/1 -> Mux/4
  Selector2/1 -> Mux/5
  Selector3/1 -> Mux/6
  Mux/1 -> Mux2/2, Scope/1, Subsystem1/1(In1)
  In5/1 -> Bus Selector1/1
  Bus Selector1/1 -> Mux1/1  "<dx>"
  Bus Selector1/2 -> Mux1/2  "<dy>"
  Bus Selector1/3 -> Mux1/3  "<dz>"
  Bus Selector1/4 -> Mux1/4  "<p>"
  Bus Selector1/5 -> Mux1/5  "<q>"
  Bus Selector1/6 -> Mux1/6  "<r>"
  Mux1/1 -> Subsystem2/1(In1)
  Mux2/1 -> MATLAB Function/1(u)
  In3/1 -> Subsystem/1(In1)
  In2/1 -> Subsystem3/1(In1)
  Bus Selector/3 -> Cast To Single/1  "<controlModePosVSOrient>"
  Cast To Single1/1 -> Mux2/3
  Subsystem1/1(Out1) -> Cast To Single1/1
  Subsystem2/1(Out1) -> Cast To Single2/1
  Data Store Read1/1 -> MATLAB Function/2(normalization)
  Data Store Read2/1 -> MATLAB Function/3("Buffer ")
  MATLAB Function/2(Buffer) -> Cast To Single3/1, Scope1/1, Data Store Write1/1
  Subsystem3/1(Out5) -> Mux2/1
  Cast To Single2/1 -> Mux2/6
  Subsystem/1(Out5) -> Mux2/5
  Cast To Single/1 -> Mux2/4
  Cast To Single3/1 -> Reshape1/1
  Demux/1 -> Scope2/1
  MATLAB Function/1(y) -> Demux/1
  Demux/2 -> Scope3/1
  Demux/3 -> Scope4/1
  Demux/4 -> Scope5/1
  Demux/5 -> Scope6/1
  Demux/6 -> Scope7/1
  Demux/7 -> Scope8/1
  Demux/8 -> Scope9/1
  Reshape1/1 -> Flip/1
  Flip/1 -> Output/1

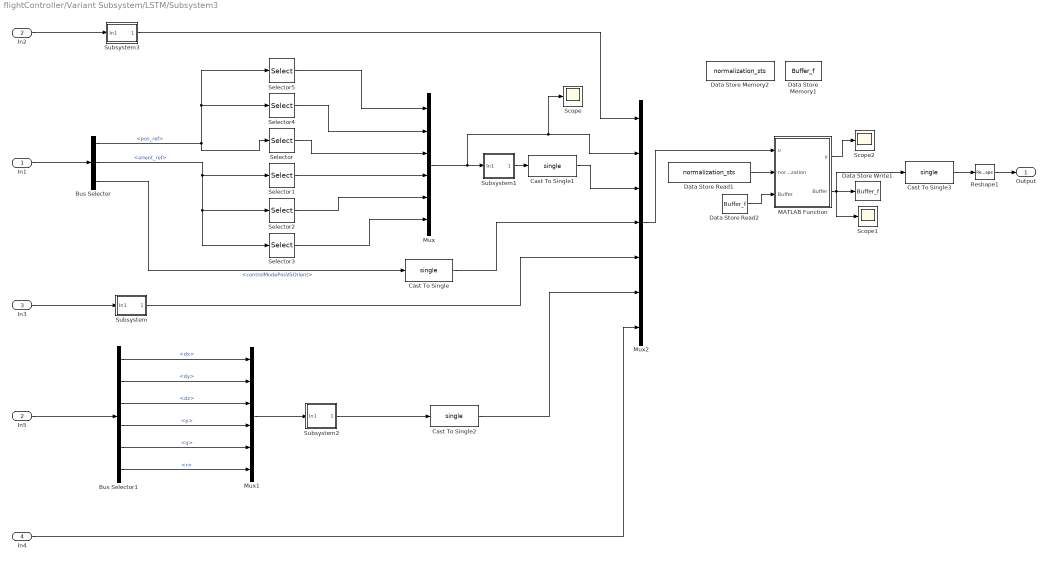
== system flightController/Variant Subsystem/LSTM/Subsystem3 ==
  In1 : Inport
  In2 : Inport  Port=2
  In3 : Inport  Port=3
  In4 : Inport  Port=4
  Bus Selector : BusSelector  OutputSignals=pos_ref,orient_ref,controlModePosVSOrient
  Bus Selector1 : BusSelector  OutputSignals=dx,dy,dz,p,q,r
  Cast To Single{,1..3} (4 alike) : DataTypeConversion  OutDataTypeStr=single
  Data Store Memory1 : DataStoreMemory  DataStoreName=Buffer_f  ReadBeforeWriteMsg=warning  WriteAfterWriteMsg=warning  WriteAfterReadMsg=warning  InitialValue=repmat(x0_f,1,delays+1)  ShowAdditionalParam=off
  Data Store Memory2 : DataStoreMemory  DataStoreName=normalization_sts  ReadBeforeWriteMsg=warning  WriteAfterWriteMsg=warning  WriteAfterReadMsg=warning  InitialValue=normalization_sts  ShowAdditionalParam=off
  Data Store Read1 : DataStoreRead  DataStoreName=normalization_sts  IndexOptions=Index vector (dialog)  Indices=1  OutputSizes=1
  Data Store Read2 : DataStoreRead  DataStoreName=Buffer_f  IndexOptions=Index vector (dialog)  Indices=1  OutputSizes=1
  Data Store Write1 : DataStoreWrite  DataStoreName=Buffer_f  IndexOptions=Index vector (dialog)  Indices=1  OutputSizes=1
  In5 : InportShadow  Port=2
  MATLAB Function : MATLAB Function  TreatAsAtomicUnit=on
  Mux : Mux  Inputs=6
  Mux1 : Mux  Inputs=6
  Mux2 : Mux  Inputs=7
      settings: DisplayOption=signals
  Reshape1 : Reshape  OutputDimensionality=Customize  OutputDimensions=[length(x0_f),delays+1]
  Scope : Scope
  Scope1 : Scope
  Scope2 : Scope
  Selector : Selector  InputPortWidth=3  IndexOptions=Index vector (dialog)  Indices=[3]  OutputSizes=1
  Selector1 : Selector  InputPortWidth=3  IndexOptions=Index vector (dialog)  Indices=[1]  OutputSizes=1
  Selector2 : Selector  InputPortWidth=3  IndexOptions=Index vector (dialog)  Indices=[3]  OutputSizes=1
  Selector3 : Selector  InputPortWidth=3  IndexOptions=Index vector (dialog)  Indices=[2]  OutputSizes=1
  Selector4 : Selector  InputPortWidth=3  IndexOptions=Index vector (dialog)  Indices=[2]  OutputSizes=1
  Selector5 : Selector  InputPortWidth=3  IndexOptions=Index vector (dialog)  Indices=[1]  OutputSizes=1
  Subsystem : Subsystem
  Subsystem1 : Subsystem
  Subsystem2 : Subsystem
  Subsystem3 : Subsystem
  Output : Outport
  wires:
  In1/1 -> Bus Selector/1
  Bus Selector/2 -> Selector3/1, Selector2/1, Selector1/1  "<orient_ref>"
  Bus Selector/1 -> Selector/1, Selector5/1, Selector4/1  "<pos_ref>"
  Selector5/1 -> Mux/1
  Selector4/1 -> Mux/2
  Selector/1 -> Mux/3
  Selector1/1 -> Mux/4
  Selector2/1 -> Mux/5
  Selector3/1 -> Mux/6
  Mux/1 -> Mux2/2, Scope/1, Subsystem1/1(In1)
  In5/1 -> Bus Selector1/1
  Bus Selector1/1 -> Mux1/1  "<dx>"
  Bus Selector1/2 -> Mux1/2  "<dy>"
  Bus Selector1/3 -> Mux1/3  "<dz>"
  Bus Selector1/4 -> Mux1/4  "<p>"
  Bus Selector1/5 -> Mux1/5  "<q>"
  Bus Selector1/6 -> Mux1/6  "<r>"
  Mux1/1 -> Subsystem2/1(In1)
  Mux2/1 -> MATLAB Function/1(u)
  MATLAB Function/1(y) -> Scope2/1
  In3/1 -> Subsystem/1(In1)
  In2/1 -> Subsystem3/1(In1)
  Bus Selector/3 -> Cast To Single/1  "<controlModePosVSOrient>"
  Cast To Single1/1 -> Mux2/3
  Subsystem1/1(Out1) -> Cast To Single1/1
  Subsystem2/1(Out1) -> Cast To Single2/1
  Data Store Read1/1 -> MATLAB Function/2(normalization)
  Data Store Read2/1 -> MATLAB Function/3("Buffer ")
  MATLAB Function/2(Buffer) -> Cast To Single3/1, Scope1/1, Data Store Write1/1
  Subsystem3/1(Out5) -> Mux2/1
  Cast To Single2/1 -> Mux2/6
  Subsystem/1(Out5) -> Mux2/5
  Cast To Single/1 -> Mux2/4
  In4/1 -> Mux2/7
  Cast To Single3/1 -> Reshape1/1
  Reshape1/1 -> Output/1

== system flightController/Variant Subsystem/ANN/Subsystem/Subsystem ==
  note: Normalizacion de Sensores
  In1 : Inport
  Bus Selector2 : BusSelector  OutputSignals=ddz,p,q,r,altitude_sonar,prs
  Mux : Mux  Inputs=6
  Subsystem1 : Subsystem
  Subsystem2 : Subsystem
  Subsystem3 : Subsystem
  Subsystem7 : Subsystem
  Subsystem8 : Subsystem
  Subsystem9 : Subsystem
  Ac_Dz : Outport
  wires:
  In1/1 -> Bus Selector2/1
  Bus Selector2/1 -> Subsystem7/1(<Ac_Dz>)  "<ddz>"
  Subsystem7/1(Ac_Dz) -> Mux/1  "Ac_Dz"
  Bus Selector2/2 -> Subsystem1/1(<Pressure Altitud>)  "<p>"
  Bus Selector2/5 -> Subsystem9/1(<Sonar Altitud>)  "<altitude_sonar>"
  Bus Selector2/6 -> Subsystem3/1(<Pressure Altitud>)  "<prs>"
  Bus Selector2/3 -> Subsystem8/1(<Pressure Altitud>)  "<q>"
  Bus Selector2/4 -> Subsystem2/1(<Pressure Altitud>)  "<r>"
  Mux/1 -> Ac_Dz/1
  Subsystem1/1(Pressure Altitud) -> Mux/2  "Gyro P"
  Subsystem8/1(Pressure Altitud) -> Mux/3  "Gyro Q"
  Subsystem2/1(Pressure Altitud) -> Mux/4  "Gyro R"
  Subsystem9/1(Sonar Altitud) -> Mux/5  "Sonar Altitud"
  Subsystem3/1(Pressure Altitud) -> Mux/6  "Pressure Altitud"

== system flightController/Variant Subsystem/ANN/Subsystem/Subsystem10 ==
  note: Normalizacion de Sensores
  note: Normalizacion_Z
  note: Normalizacion de ref_Z
  note: Normalizacion_DZ
  note: Normalizacion_Acel_Z
  note: Normalizacion de ref_DZ
  In1 : Inport
  Bus Creator : BusCreator  Inputs=8
  Bus Selector : BusSelector  OutputSignals=Z,Dz,Z_r,Dz_r,Ac_Dz,Sonar Altitud,Pressure Altitud,Acceleracion Z
  Subsystem : Subsystem
  Subsystem2 : Subsystem
  Subsystem3 : Subsystem
  Subsystem4 : Subsystem
  Subsystem6 : Subsystem
  Subsystem7 : Subsystem
  Subsystem8 : Subsystem
  Subsystem9 : Subsystem
  Output : Outport
  wires:
  In1/1 -> Bus Selector/1
  Bus Selector/6 -> Subsystem9/1(<Sonar Altitud>)  "<Sonar Altitud>"
  Subsystem3/1(Z) -> Bus Creator/1
  Subsystem/1(Z_r) -> Bus Creator/3
  Subsystem9/1(Sonar Altitud) -> Bus Creator/6
  Subsystem6/1(Acceleracion Z) -> Bus Creator/8
  Bus Selector/1 -> Subsystem3/1(<Z>)  "<Z>"
  Subsystem7/1(Ac_Dz) -> Bus Creator/5
  Subsystem2/1(Dz_r) -> Bus Creator/4
  Bus Selector/3 -> Subsystem/1(<Z_r>)  "<Z_r>"
  Bus Selector/2 -> Subsystem4/1(<dz>)  "<Dz>"
  Subsystem4/1(Dz) -> Bus Creator/2
  Bus Selector/5 -> Subsystem7/1(<Ac_Dz>)  "<Ac_Dz>"
  Bus Creator/1 -> Output/1
  Subsystem8/1(Pressure Altitud) -> Bus Creator/7
  Bus Selector/4 -> Subsystem2/1(<Dz_r>)  "<Dz_r>"
  Bus Selector/7 -> Subsystem8/1(<Pressure Altitud>)  "<Pressure Altitud>"
  Bus Selector/8 -> Subsystem6/1(<Acel_z>)  "<Acceleracion Z>"

== system flightController/Variant Subsystem/ANN/Subsystem/Subsystem11 ==
  note: Normalizacion de ref_DZ
  note: Normalizacion_Z
  note: Normalizacion de ref_Z
  note: Normalizacion_Acel_Z
  note: Normalizacion de Sensores
  note: Normalizacion_DZ
  In1 : Inport
  Bus Creator : BusCreator  Inputs=8
  Bus Selector1 : BusSelector  OutputSignals=Z,Dz,Z_r,Dz_r,Ac_Dz,Sonar Altitud,Pressure Altitud,Acceleracion Z
  Subsystem : Subsystem
  Subsystem2 : Subsystem
  Subsystem3 : Subsystem
  Subsystem4 : Subsystem
  Subsystem6 : Subsystem
  Subsystem7 : Subsystem
  Subsystem8 : Subsystem
  Subsystem9 : Subsystem
  Output : Outport
  wires:
  Bus Selector1/4 -> Subsystem2/1(<Dz_r>)  "<Dz_r>"
  Bus Selector1/2 -> Subsystem4/1(<dz>)  "<Dz>"
  Bus Selector1/8 -> Subsystem6/1(<Acel_z>)  "<Acceleracion Z>"
  Bus Selector1/1 -> Subsystem3/1(<Z>)  "<Z>"
  In1/1 -> Bus Selector1/1
  Bus Selector1/7 -> Subsystem8/1(<Pressure Altitud>)  "<Pressure Altitud>"
  Subsystem8/1(Pressure Altitud) -> Bus Creator/7
  Subsystem4/1(Dz) -> Bus Creator/2
  Subsystem7/1(Ac_Dz) -> Bus Creator/5
  Bus Selector1/6 -> Subsystem9/1(<Sonar Altitud>)  "<Sonar Altitud>"
  Subsystem9/1(Sonar Altitud) -> Bus Creator/6
  Subsystem2/1(Dz_r) -> Bus Creator/4
  Subsystem6/1(Acceleracion Z) -> Bus Creator/8
  Bus Creator/1 -> Output/1
  Bus Selector1/5 -> Subsystem7/1(<Ac_Dz>)  "<Ac_Dz>"
  Bus Selector1/3 -> Subsystem/1(<Z_r>)  "<Z_r>"
  Subsystem3/1(Z) -> Bus Creator/1
  Subsystem/1(Z_r) -> Bus Creator/3

== system flightController/Variant Subsystem/ANN/Subsystem/Subsystem12 ==
  note: Normalizacion_DZ
  note: Normalizacion de Sensores
  note: Normalizacion_Acel_Z
  note: Normalizacion de ref_Z
  note: Normalizacion_Z
  note: Normalizacion de ref_DZ
  In1 : Inport
  Bus Creator : BusCreator  Inputs=8
  Bus Selector1 : BusSelector  OutputSignals=Z,Dz,Z_r,Dz_r,Ac_Dz,Sonar Altitud,Pressure Altitud,Acceleracion Z
  Subsystem : Subsystem
  Subsystem2 : Subsystem
  Subsystem3 : Subsystem
  Subsystem4 : Subsystem
  Subsystem6 : Subsystem
  Subsystem7 : Subsystem
  Subsystem8 : Subsystem
  Subsystem9 : Subsystem
  Output : Outport
  wires:
  Subsystem/1(Z_r) -> Bus Creator/3
  Subsystem3/1(Z) -> Bus Creator/1
  Bus Selector1/3 -> Subsystem/1(<Z_r>)  "<Z_r>"
  Bus Selector1/5 -> Subsystem7/1(<Ac_Dz>)  "<Ac_Dz>"
  Bus Creator/1 -> Output/1
  Subsystem6/1(Acceleracion Z) -> Bus Creator/8
  Subsystem2/1(Dz_r) -> Bus Creator/4
  Subsystem9/1(Sonar Altitud) -> Bus Creator/6
  Bus Selector1/6 -> Subsystem9/1(<Sonar Altitud>)  "<Sonar Altitud>"
  Subsystem7/1(Ac_Dz) -> Bus Creator/5
  Subsystem4/1(Dz) -> Bus Creator/2
  Subsystem8/1(Pressure Altitud) -> Bus Creator/7
  Bus Selector1/7 -> Subsystem8/1(<Pressure Altitud>)  "<Pressure Altitud>"
  In1/1 -> Bus Selector1/1
  Bus Selector1/1 -> Subsystem3/1(<Z>)  "<Z>"
  Bus Selector1/8 -> Subsystem6/1(<Acel_z>)  "<Acceleracion Z>"
  Bus Selector1/2 -> Subsystem4/1(<dz>)  "<Dz>"
  Bus Selector1/4 -> Subsystem2/1(<Dz_r>)  "<Dz_r>"

== system flightController/Variant Subsystem/ANN/Subsystem/Subsystem13 ==
  note: Acel_Z
  note: Normalizacion_DZ
  note: Normalizacion_Z
  note: Normalizacion_Acel_Z
  note: Normalizacion_YAW
  note: Normalizacion_ROLL
  note: Normalizacion_PITCH
  note: Normalizacion_P
  note: Normalizacion_Q
  note: Normalizacion_R
  note: Acel_P
  note: Normalizacion_Acel_P
  note: Acel_Q
  note: Normalizacion_Acel_Q
  note: Acel_R
  note: Normalizacion_Acel_R
  In1 : Inport
  Bus Selector1 : BusSelector  OutputSignals=Z,yaw,roll,pitch,dz,p,q,r
  Mux : Mux  Inputs=7
  Mux1 : Mux  Inputs=1
  Subsystem1 : Subsystem  Commented=on
  Subsystem10 : Subsystem
  Subsystem11 : Subsystem  Commented=on
  Subsystem12 : Subsystem  Commented=on
  Subsystem13 : Subsystem  Commented=on
  Subsystem14 : Subsystem  Commented=on
  Subsystem15 : Subsystem  Commented=on
  Subsystem16 : Subsystem  Commented=on
  Subsystem2 : Subsystem
  Subsystem3 : Subsystem
  Subsystem4 : Subsystem
  Subsystem5 : Subsystem
  Subsystem6 : Subsystem
  Subsystem7 : Subsystem
  Subsystem8 : Subsystem
  Subsystem9 : Subsystem
  Pos_Norm : Outport
  Acceleracion Pos : Outport  Port=2
  wires:
  Bus Selector1/1 -> Subsystem3/1(<Z>)  "<Z>"
  Bus Selector1/5 -> Subsystem4/1(<dz>), Subsystem5/1(In1)  "<dz>"
  Subsystem5/1(<Acel_Z>) -> Subsystem6/1(<Acel_z>)
  In1/1 -> Bus Selector1/1
  Bus Selector1/2 -> Subsystem1/1(<Z>)  "<yaw>"
  Bus Selector1/6 -> Subsystem11/1(In1), Subsystem8/1(<dz>)  "<p>"
  Bus Selector1/7 -> Subsystem13/1(In1), Subsystem9/1(<Z>)  "<q>"
  Bus Selector1/8 -> Subsystem15/1(In1), Subsystem10/1(<Z>)  "<r>"
  Mux/1 -> Pos_Norm/1
  Subsystem3/1(Z) -> Mux/1  "Z"
  Mux1/1 -> Acceleracion Pos/1
  Subsystem6/1(Acceleracion Z) -> Mux1/1  "Acceleracion Z"
  Subsystem11/1(<Acel_Z>) -> Subsystem12/1(<Acel_z>)
  Subsystem12/1(Acceleracion Z) -> ?  "Acceleracion Z"
  Subsystem13/1(<Acel_Z>) -> Subsystem14/1(<Acel_z>)
  Subsystem14/1(Acceleracion Z) -> ?  "Acceleracion Z"
  Subsystem15/1(<Acel_Z>) -> Subsystem16/1(<Acel_z>)
  Subsystem16/1(Acceleracion Z) -> ?  "Acceleracion Z"
  Bus Selector1/3 -> Subsystem2/1(<Z>)  "<roll>"
  Bus Selector1/4 -> Subsystem7/1(<Z>)  "<pitch>"
  Subsystem2/1(Z) -> Mux/2  "Z"
  Subsystem7/1(Z) -> Mux/3  "Z"
  Subsystem4/1(Dz) -> Mux/4  "Dz"
  Subsystem8/1(Dz) -> Mux/5  "Dz"
  Subsystem9/1(Z) -> Mux/6  "Z"
  Subsystem10/1(Z) -> Mux/7  "Z"

== system flightController/Variant Subsystem/ANN/Subsystem/Subsystem3 ==
  note: Normalizacion de ref_Z
  note: ref_DZ
  note: Normalizacion de ref_DZ
  note: Normalizacion de ref_YAW
  note: Normalizacion de ref_ROLL
  note: Normalizacion de ref_PITCH
  note: Normalizacion de ref_P
  note: Normalizacion de ref_Q
  note: Normalizacion de ref_R
  In1 : Inport
  Bus Selector : BusSelector  OutputSignals=pos_ref,orient_ref
  Demux : Demux
  Mux : Mux
  Mux1 : Mux  Inputs=3
  Mux2 : Mux  Inputs=1
  Selector : Selector  InputPortWidth=3  IndexOptions=Index vector (dialog)  Indices=[3]  OutputSizes=1
  Selector1 : Selector  InputPortWidth=3  IndexOptions=Index vector (dialog)  Indices=[1]  OutputSizes=1
  Selector2 : Selector  InputPortWidth=3  IndexOptions=Index vector (dialog)  Indices=[3]  OutputSizes=1
  Selector3 : Selector  InputPortWidth=3  IndexOptions=Index vector (dialog)  Indices=[2]  OutputSizes=1
  Subsystem : Subsystem
  Subsystem1 : Subsystem
  Subsystem2 : Subsystem
  Subsystem3 : Subsystem  Commented=on
  Subsystem4 : Subsystem
  Subsystem5 : Subsystem
  Subsystem6 : Subsystem  Commented=on
  Subsystem7 : Subsystem  Commented=on
  Subsystem8 : Subsystem  Commented=on
  Z_r : Outport
  Dz_r : Outport  Port=2
  wires:
  Bus Selector/1 -> Selector/1  "<pos_ref>"
  Selector/1 -> Mux/1, Subsystem/1(<Z_r>)
  In1/1 -> Bus Selector/1
  Bus Selector/2 -> Selector2/1, Selector3/1, Selector1/1  "<orient_ref>"
  Selector1/1 -> Mux/2, Subsystem3/1(<Z_r>)
  Selector2/1 -> Mux/3, Subsystem4/1(<Z_r>)
  Selector3/1 -> Mux/4, Subsystem5/1(<Z_r>)
  Mux/1 -> Subsystem1/1(In1)
  Subsystem1/1(Out1) -> Demux/1
  Demux/1 -> Subsystem2/1(<Dz_r>)
  Demux/2 -> Subsystem6/1(<Dz_r>)
  Demux/3 -> Subsystem7/1(<Dz_r>)
  Demux/4 -> Subsystem8/1(<Dz_r>)
  Subsystem/1(Z_r) -> Mux1/1  "Z_r"
  Mux1/1 -> Z_r/1
  Subsystem2/1(Dz_r) -> Mux2/1  "Dz_r"
  Subsystem6/1(Dz_r) -> ?  "Dz_r"
  Subsystem7/1(Dz_r) -> ?  "Dz_r"
  Subsystem8/1(Dz_r) -> ?  "Dz_r"
  Mux2/1 -> Dz_r/1
  Subsystem5/1(Z_r) -> Mux1/3  "Z_r"
  Subsystem4/1(Z_r) -> Mux1/2  "Z_r"

== system flightController/Variant Subsystem/ANN/Subsystem2/Subsystem ==
  In1 : Inport
  Bus Selector2 : BusSelector  OutputSignals=ddx,ddy,ddz,p,q,r,altitude_sonar,prs,vbat_V,vbat_percentage
  Cast To Single : DataTypeConversion  OutDataTypeStr=single
  Mux : Mux  Inputs=10
  Scope : Scope
  Out5 : Outport
  wires:
  In1/1 -> Bus Selector2/1
  Bus Selector2/1 -> Mux/1  "<ddx>"
  Bus Selector2/2 -> Mux/2  "<ddy>"
  Bus Selector2/3 -> Mux/3  "<ddz>"
  Bus Selector2/4 -> Mux/4  "<p>"
  Bus Selector2/5 -> Mux/5  "<q>"
  Bus Selector2/6 -> Mux/6  "<r>"
  Bus Selector2/7 -> Mux/7  "<altitude_sonar>"
  Bus Selector2/8 -> Mux/8  "<prs>"
  Bus Selector2/9 -> Mux/9  "<vbat_V>"
  Mux/1 -> Scope/1, Out5/1
  Bus Selector2/10 -> Cast To Single/1  "<vbat_percentage>"
  Cast To Single/1 -> Mux/10

== system flightController/Variant Subsystem/ANN/Subsystem2/Subsystem1 ==
  In1 : Inport
  Constant1 : Constant  Value=Ts
  Delay1 : Delay  DelayLength=1  InitialCondition=0
  Divide1 : Product  Inputs=*/
  Sum1 : Sum  Inputs=|+-
  Out1 : Outport
  wires:
  In1/1 -> Delay1/1, Sum1/1
  Constant1/1 -> Divide1/2
  Sum1/1 -> Divide1/1
  Delay1/1 -> Sum1/2
  Divide1/1 -> Out1/1
